simulink model "APM_control_scheme_22b"  (R2022b)
settings: Solver=VariableStepAuto  StartTime=0.0  StopTime=10.0  RelTol=1e-3
InitFcn:
  | init_APM
undefined symbols (not defined in the file or in its folder): pa
settings Model: Creator=HQ03  LastModifiedBy=HQ03

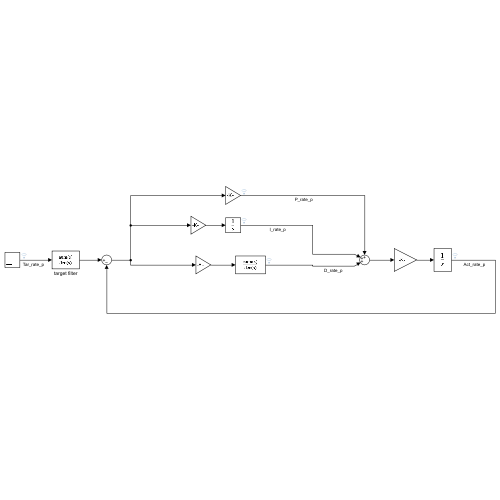
[thumbnail: Simulink's stored preview of the top-level diagram]
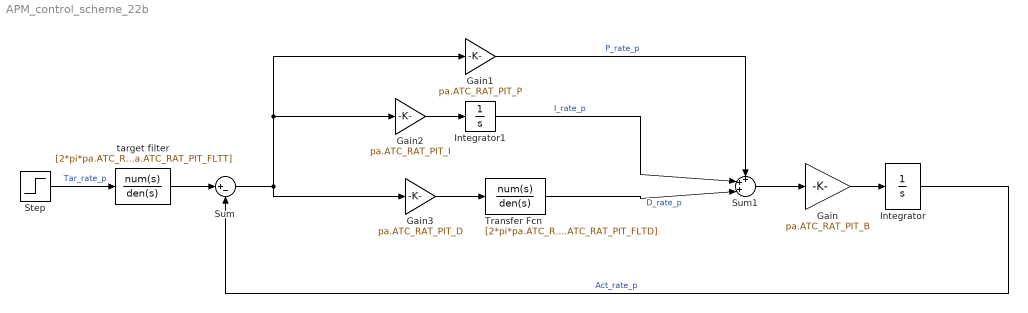
== system APM_control_scheme_22b ==
  Gain : Gain  Gain=pa.ATC_RAT_PIT_B
  Gain1 : Gain  Gain=pa.ATC_RAT_PIT_P
  Gain2 : Gain  Gain=pa.ATC_RAT_PIT_I
  Gain3 : Gain  Gain=pa.ATC_RAT_PIT_D
  Integrator : Integrator
  Integrator1 : Integrator
  Step : Step  SampleTime=0
  Sum : Sum  Inputs=|+-
  Sum1 : Sum  Inputs=+++|
  Transfer Fcn : TransferFcn  Numerator=[2*pi*pa.ATC_RAT_PIT_FLTD 0]  Denominator=[1 2*pi*pa.ATC_RAT_PIT_FLTD]
  target filter : TransferFcn  Numerator=[2*pi*pa.ATC_RAT_PIT_FLTT]  Denominator=[1 2*pi*pa.ATC_RAT_PIT_FLTT]
  wires:
  Gain/1 -> Integrator/1
  Step/1 -> target filter/1  "Tar_rate_p"
  Integrator/1 -> Sum/2  "Act_rate_p"
  target filter/1 -> Sum/1
  Sum1/1 -> Gain/1
  Sum/1 -> Gain1/1, Gain2/1, Gain3/1
  Gain1/1 -> Sum1/1  "P_rate_p"
  Gain2/1 -> Integrator1/1
  Gain3/1 -> Transfer Fcn/1
  Integrator1/1 -> Sum1/2  "I_rate_p"
  Transfer Fcn/1 -> Sum1/3  "D_rate_p"
